simulink model "adrc_pid"  (Simulink 7.6)
settings: Solver=ode45  StartTime=0.0  StopTime=10.0  RelTol=1e-3
values from neighbouring files (symbols this model uses):
  K = [9.375  -6.25; -8.125  8.75]    [PP2013428.mat]
libraries: opclib x5, ADRC x2, simulink x2
settings Model: Creator=Administrator  LastModifiedBy=Administrator

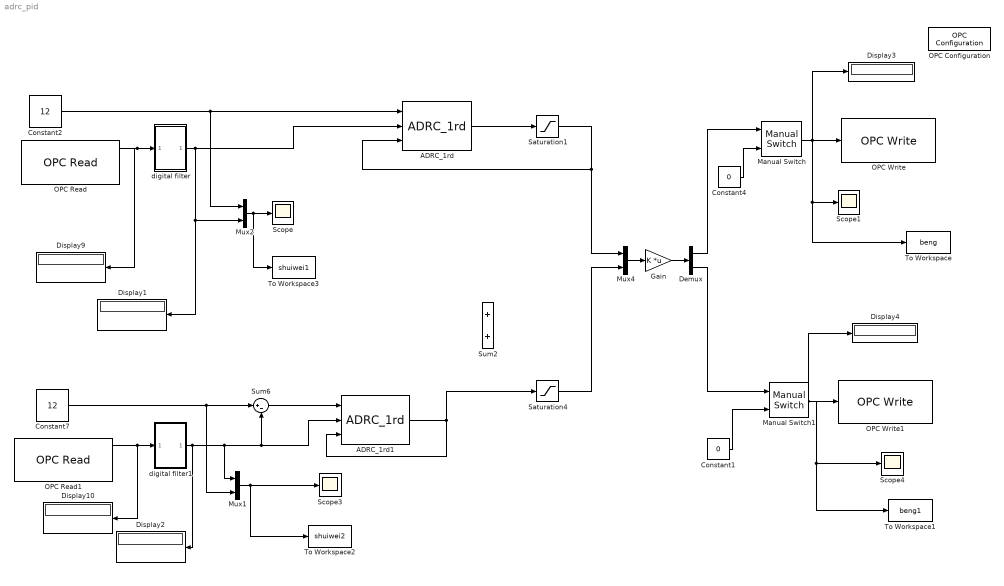
== system adrc_pid ==
  ADRC_1rd : ADRC/ADRC/ADRC_1rd/ADRC_1rd  SystemSampleTime=-1  r0=0.01  h=0.1  B01=10  B02=20  r=8
  ADRC_1rd1 : ADRC/ADRC/ADRC_1rd/ADRC_1rd  SystemSampleTime=-1  r0=0.01  h=0.1  B01=10  B02=20  r=8
  Constant1 : Constant  Value=0
  Constant2 : Constant  Value=12
  Constant4 : Constant  Value=0
  Constant7 : Constant  Value=12
  Demux : Demux  Outputs=2
  Display{1..4,9..10} (6 alike) : Display
  Gain : Gain  Gain=K  Multiplication=Matrix(K*u)
  Manual Switch : simulink/Signal Routing/Manual Switch  SystemSampleTime=-1  sw=0  action=0  varsize=off
  Manual Switch1 : simulink/Signal Routing/Manual Switch  SystemSampleTime=-1  sw=0  action=0  varsize=off
  Mux1 : Mux  Inputs=2
  Mux2 : Mux  Inputs=2
  Mux4 : Mux  Inputs=2
  OPC Configuration : opclib/OPC Configuration  opcServers=localhost/OPCServer.WinCC/10  errMissingItems=Error  errReadWrite=Warn  errShutdown=Error  errRTViolation=None  rtEnable=on  speedup=1  showLatency=off  beingUsed=on
  OPC Read : opclib/OPC Read  serverHost=localhost  serverID=OPCServer.WinCC  itemIDs=shuiwei1  readMode=Synchronous (cache)  dataType=double  updateRate=0.01  showQual=on  showTS=on  tsMode=Seconds since start
  OPC Read1 : opclib/OPC Read  serverHost=localhost  serverID=OPCServer.WinCC  itemIDs=shuiwei2  readMode=Synchronous (cache)  dataType=double  updateRate=0.5  showQual=on  showTS=on  tsMode=Seconds since start
  OPC Write : opclib/OPC Write  serverHost=localhost  serverID=OPCServer.WinCC  itemIDs=beng1  writeMode=Synchronous  updateRate=0
  OPC Write1 : opclib/OPC Write  serverHost=localhost  serverID=OPCServer.WinCC  itemIDs=beng2  writeMode=Synchronous  updateRate=0
  Saturation1 : Saturate  UpperLimit=100  LowerLimit=0
  Saturation4 : Saturate  UpperLimit=100  LowerLimit=0
  Scope{,1,3..4} (4 alike) : Scope
      Scope settings: TimeRange=1000  YMin=0  YMax=20  SaveName=shuiwei4  DataFormat=Array
      Scope1 settings: TimeRange=1000  YMin=82.5  YMax=89.5  SaveName=shuiwei  DataFormat=Array
      Scope3 settings: TimeRange=1000  YMin=0  YMax=20  SaveName=shuiwei5  DataFormat=Array
      Scope4 settings: TimeRange=1000  YMin=0  YMax=100  SaveName=shuiwei3  DataFormat=Array
  Sum2 : Sum
  Sum6 : Sum  Inputs=|+-
  To Workspace : ToWorkspace  VariableName=beng  SampleTime=0.5  SaveFormat=Array
  To Workspace1 : ToWorkspace  VariableName=beng1  SampleTime=0.5  SaveFormat=Array
  To Workspace2 : ToWorkspace  VariableName=shuiwei2  SampleTime=0.5  SaveFormat=Array
  To Workspace3 : ToWorkspace  VariableName=shuiwei1  SampleTime=0.5  SaveFormat=Array
  digital filter : Subsystem
  digital filter1 : Subsystem
  wires:
  Constant2/1 -> Mux2/1, ADRC_1rd/1
  Manual Switch/1 -> OPC Write/1, Display3/1, Scope1/1, To Workspace/1
  Constant4/1 -> Manual Switch/2
  Constant7/1 -> Sum6/1, Mux1/2
  Sum6/1 -> ADRC_1rd1/1
  Manual Switch1/1 -> OPC Write1/1, Display4/1, Scope4/1, To Workspace1/1
  OPC Read1/1 -> Display10/1, digital filter1/1(In1)
  OPC Read/1 -> Display9/1, digital filter/1(In1)
  Constant1/1 -> Manual Switch1/2
  Mux2/1 -> Scope/1, To Workspace3/1
  Mux1/1 -> Scope3/1, To Workspace2/1
  digital filter/1(Out1) -> Display1/1, Mux2/2, ADRC_1rd/2
  digital filter1/1(Out1) -> Mux1/1, Sum6/2, ADRC_1rd1/2, Display2/1
  ADRC_1rd/1 -> Saturation1/1
  ADRC_1rd1/1 -> ADRC_1rd1/3, Saturation4/1
  Saturation1/1 -> Mux4/1, ADRC_1rd/3
  Saturation4/1 -> Mux4/2
  Mux4/1 -> Gain/1
  Gain/1 -> Demux/1
  Demux/1 -> Manual Switch/1
  Demux/2 -> Manual Switch1/1

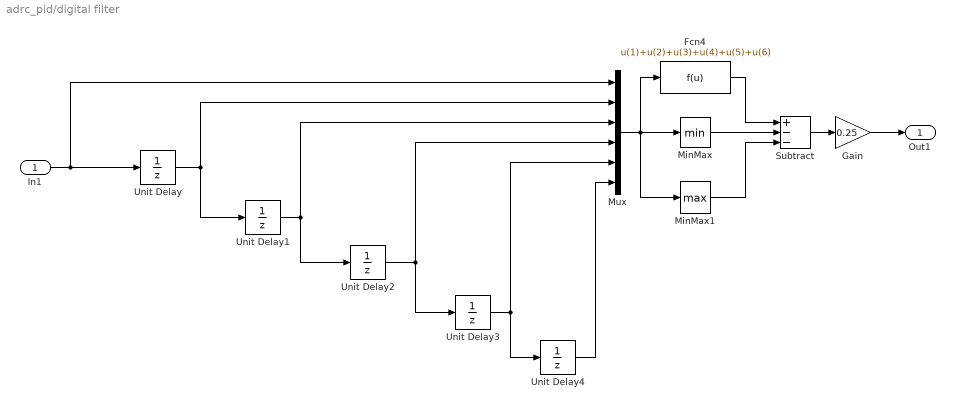
== system adrc_pid/digital filter ==
  In1 : Inport
  Fcn4 : Fcn  Expr=u(1)+u(2)+u(3)+u(4)+u(5)+u(6)  SampleTime=0.5
  Gain : Gain  Gain=0.25
  MinMax : MinMax
  MinMax1 : MinMax  Function=max
  Mux : Mux  Inputs=6
  Subtract : Sum  Inputs=+--
  Unit Delay{,1..4} (5 alike) : UnitDelay  SampleTime=0.5
  Out1 : Outport
  wires:
  Unit Delay/1 -> Mux/2, Unit Delay1/1
  Unit Delay1/1 -> Mux/3, Unit Delay2/1
  Unit Delay2/1 -> Mux/4, Unit Delay3/1
  In1/1 -> Unit Delay/1, Mux/1
  Unit Delay3/1 -> Mux/5, Unit Delay4/1
  Mux/1 -> Fcn4/1, MinMax/1, MinMax1/1
  Fcn4/1 -> Subtract/1
  MinMax/1 -> Subtract/2
  MinMax1/1 -> Subtract/3
  Subtract/1 -> Gain/1
  Unit Delay4/1 -> Mux/6
  Gain/1 -> Out1/1

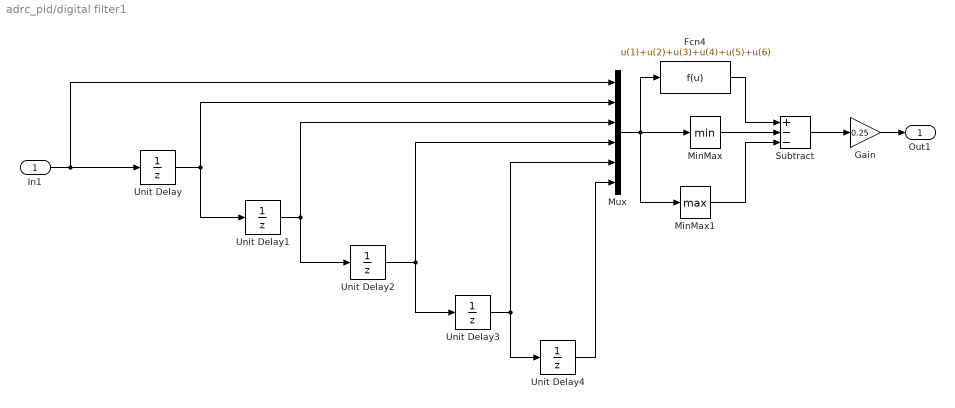
== system adrc_pid/digital filter1 ==
  In1 : Inport
  Fcn4 : Fcn  Expr=u(1)+u(2)+u(3)+u(4)+u(5)+u(6)  SampleTime=0.5
  Gain : Gain  Gain=0.25
  MinMax : MinMax
  MinMax1 : MinMax  Function=max
  Mux : Mux  Inputs=6
  Subtract : Sum  Inputs=+--
  Unit Delay{,1..4} (5 alike) : UnitDelay  SampleTime=0.5
  Out1 : Outport
  wires:
  Gain/1 -> Out1/1
  Unit Delay4/1 -> Mux/6
  Subtract/1 -> Gain/1
  MinMax1/1 -> Subtract/3
  MinMax/1 -> Subtract/2
  Fcn4/1 -> Subtract/1
  Mux/1 -> MinMax1/1, MinMax/1, Fcn4/1
  Unit Delay3/1 -> Unit Delay4/1, Mux/5
  In1/1 -> Mux/1, Unit Delay/1
  Unit Delay2/1 -> Unit Delay3/1, Mux/4
  Unit Delay1/1 -> Unit Delay2/1, Mux/3
  Unit Delay/1 -> Unit Delay1/1, Mux/2
